simulink library "libSimulators"  (R2015a)
settings: Solver=ode45  StartTime=0.0  StopTime=10.0  RelTol=1e-3
settings Model: CovSFcnEnable=off  Creator=jcardena  LastModifiedBy=jcardena
settings DebuggingCC: SolverPrmCheckMsg=warning

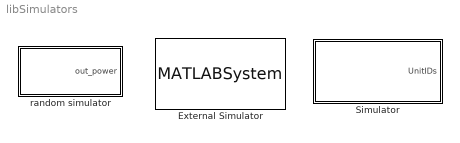
== system libSimulators ==
  External Simulator : MATLABSystem  System=slexVarSizeMATLABSystemGetDBIDsSysObj  Condition=%20151209%  N=100  db_name=WaterHeaters  db_username=sw_waterheaters  db_password=unb.sql.2015
      mask Type: slexVarSizeMATLABSystemGetDBIDsSysObj
      mask Display:
      | disp('slexVarSizeMATLABSystemGetDBIDsSysObj');
      | port_label('output',1,'Output');
      | port_label('output',2,'unitIDs');
  Simulator : Subsystem  mask(Simulator mask){unitIDs=0, searchString='%20151209%', db_name=HeatingUnits, db_username=sw_waterheaters, db_password=unb.sql.2015, msgError_edit=Connection successful}
      mask prompts: searchString "Unit Name contains"; db_name "Database name"; db_username "username"; db_password "password"; msgError_edit "Status"
      mask TypeOptions db_name: WaterHeaters | HeatingUnits | powerMeters
      mask TypeOptions db_username: sw_waterheaters | sw_ETS | sw_powermeters
      mask DialogControl msgGroupVar Prompt: Test Database Connection
      mask DialogControl db_connect_btn Prompt: Test
      mask DialogControl db_connect_btn Callback:
      | db_username = get_param(gcb, 'db_username');
      | db_password = get_param(gcb, 'db_password');
      | login.username = db_username; login.password = db_password;
      | db_name = get_param(gcb, 'db_name');
      | conn = open_sql_conn(db_name, login);
      | if (isempty(conn))
      | 
      |     set_param(gcb,'msgError_edit','Error in the connection');
      | else
      |     set_param(gcb,'msgError_edit','Connection successful');
      |     close(conn);
      | end
      | clear conn;
      mask Display: disp(['Database\n' get_param(gcb, 'db_name')])
  random simulator : Subsystem  mask(Simulator type){rated_power=6000, N=1}
      mask prompts: rated_power "Rated Power"; N "Number of  samples"
      mask help: Simulator description

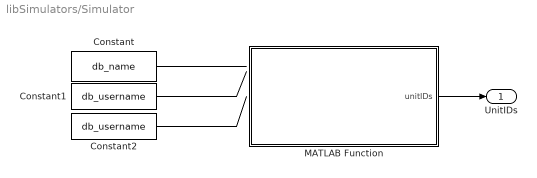
== system libSimulators/Simulator ==
  Constant : Constant  Value=db_name
  Constant1 : Constant  Value=db_username
  Constant2 : Constant  Value=db_username
  MATLAB Function : MATLAB Function  TreatAsAtomicUnit=on
  UnitIDs : Outport  OutDataTypeStr=double
  wires:
  MATLAB Function/1(unitIDs) -> UnitIDs/1
  Constant/1 -> ?
  Constant1/1 -> ?
  Constant2/1 -> ?

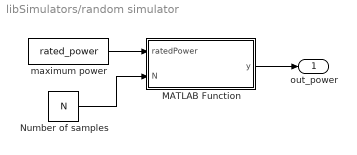
== system libSimulators/random simulator ==
  MATLAB Function : MATLAB Function  TreatAsAtomicUnit=on
  Number of samples : Constant  Value=N
  maximum power : Constant  Value=rated_power
  out_power : Outport
  wires:
  MATLAB Function/1(y) -> out_power/1
  maximum power/1 -> MATLAB Function/1(ratedPower)
  Number of samples/1 -> MATLAB Function/2(N)

== matlab function libSimulators/Simulator/MATLAB Function ==
  data: unitIDs output
function unitIDs   = db_get_unitids
%#codegen
coder.extrinsic('gcb');
coder.extrinsic('get_param');
coder.extrinsic('getUnitIds');

db_name = get_param(gcb, 'db_name');
db_username = get_param(gcb, 'db_username');
db_password = get_param(gcb, 'db_password');
unitIDs  = getUnitIds (db_name, db_username, db_password);
end

function unitIDs   = getUnitIds (db_name,db_username, db_password);
login.username = db_username; 
login.password = db_password;

    
conn = open_sql_conn(db_name, login);

searchStr = get_param(gcb, 'searchString');

%% TO DO: too particular. More general code should be implemented here
if (strcmpi('WaterHeaters',db_name))
    id_column_name = 'WaterHeaterID';
    name_column_name = 'WaterHeaterName';
end

if (strcmpi('heatingUnits',db_name))
    id_column_name = 'ETSID';
    name_column_name = 'ETSName';
end

if (strcmpi('powerMeters',db_name))
    id_column_name = 'MeterID';
    name_column_name = 'MeterName';
end

%%
unitIDs = fetch(conn, [' SELECT 	' id_column_name...
    ,' FROM ', db_name, ' WHERE ', name_column_name, ' LIKE ', searchStr  ]); 
%Close database connection.
close(conn);
end

== matlab function libSimulators/random simulator/MATLAB Function ==
  data: ratedPower input; y output double [0..rated_power]; N input size=1
function y = random_power(ratedPower, N)
%#codegen

y = randi(ratedPower,[1,N]);
